simulink model "svpwm_matlab"  (Simulink 7.4)
settings: Solver=ode45  StartTime=0.0  StopTime=0.4  RelTol=1e-3
InitFcn:
  | fc_bus=50;
  | car_freq=4500;
  | TsMLIV=20e-6;
  | Ts=2e-6;
undefined symbols (not defined in the file): DiscIntNeverNeededParam
libraries: powerlib x15, powerlib_extras x3, AC2DriveInternalModels x2
settings Model: Creator=Kashif  LastModifiedBy=Kashif

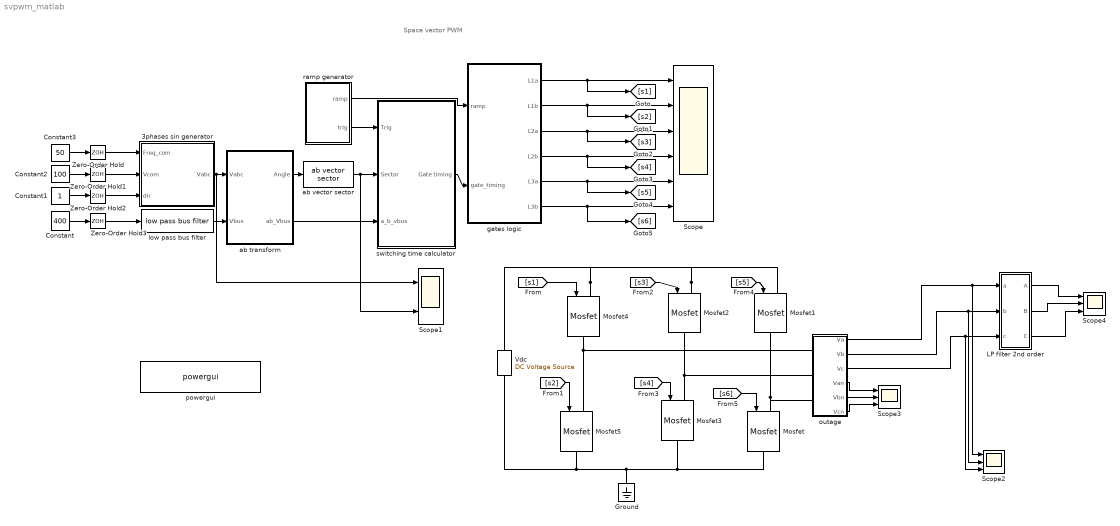
== system svpwm_matlab ==
  note: Space vector PWM
  3phases sin generator : Subsystem  AncestorBlock=AC2DriveInternalModels/SVM generator/3phases sin generator
  Constant : Constant  Value=400  OutDataType=fixdt(1, 16)  OutScaling=2^0
  Constant1 : Constant  OutDataType=fixdt(1, 16)  OutScaling=2^0
  Constant2 : Constant  Value=100  OutDataType=fixdt(1, 16)  OutScaling=2^0
  Constant3 : Constant  Value=50  OutDataType=fixdt(1, 16)  OutScaling=2^0
  Ground : powerlib/Elements/Ground  DialogController=POWERSYS.PowerSysDialog  PhysicalDomain=powersysdomain  SubClassName=unknown  LeftPortType=p1  RightPortType=p1  LConnTagsString=a
  LP filter 2nd order : Subsystem  mask{cutoff_frequency=200, damping_factor=0.707}
      mask prompts: cutoff_frequency "Cut off frequency"; damping_factor "Damping Factor"
  Mosfet{,1..5} (6 alike) : powerlib/Power Electronics/Mosfet  DialogController=POWERSYS.PowerSysDialog  SystemSampleTime=-1  Ron=0.1  Lon=0  Rd=0.01  Vfd=0  IC=0  Rs=1e5  Cs=inf  Measurements=off
  Scope : Scope  NumInputPorts=6
      settings: YMin=-5~-5~-5~-5~-5~-5  YMax=5~5~5~5~5~5  MaxDataPoints=5000000  SampleInput=on  SampleTime=2e-6
  Scope1 : Scope  NumInputPorts=2
      settings: YMin=-5~-5  YMax=5~5  MaxDataPoints=5000000  SampleInput=on  SampleTime=2e-6
  Scope2 : Scope  NumInputPorts=3
      settings: YMin=-450~-5~-5  YMax=450~5~5  SaveName=Line_voltages  MaxDataPoints=5000000  SampleInput=on  SampleTime=2e-6
  Scope3 : Scope  NumInputPorts=3
      settings: YMin=-5~-5~-5  YMax=5~5~5  SaveName=Neutral_voltages  MaxDataPoints=5000000  SampleInput=on  SampleTime=2e-6
  Scope4 : Scope  NumInputPorts=3
      settings: YMin=-450~-450~-450  YMax=450~450~450  SaveName=Filtered_voltages  MaxDataPoints=5000000  SampleInput=on  SampleTime=2e-6
  Vdc : powerlib/Electrical Sources/DC Voltage Source  DialogController=POWERSYS.PowerSysDialog  SystemSampleTime=-1  Amplitude=400  Measurements=None
  Zero-Order Hold{,1..3} (4 alike) : ZeroOrderHold  SampleTime=TsMLIV
  ab transform : Subsystem  AncestorBlock=AC2DriveInternalModels/SVM generator/ab transform
  ab vector sector : AC2DriveInternalModels/SVM generator/ab vector sector  SystemSampleTime=-1
  gates logic : Subsystem  AncestorBlock=AC2DriveInternalModels/SVM generator/gates logic
  low pass bus filter : AC2DriveInternalModels/SVM generator/low pass bus filter  SystemSampleTime=-1
  outage : Subsystem
  powergui : powerlib/powergui  Priority=1  SystemSampleTime=-1  SimulationMode=Discrete  SampleTime=2e-6  frequency=60  SPID=off  DisableSnubberDevices=off  DisableRonSwitches=off  DisableVfSwitches=off  SwTol=0  Interpol=off  frequencyindice=0  echomessages=off  HookPort=off  DisplayEquations=off  FunctionMessages=off  EnableUseOfTLC=off  x0status=blocks  RestoreLinks=warning  Frange=[0:2:500]  Ylog=off  Xlog=on  ShowGrid=off  save=off  variable=ZData  structure=Line_voltages  ZoomFFT=off  StartTime=0.04  cycles=1  DisplayStyle=2  fundamental=50  FreqAxis=off  MaxFrequency=10000  frequencyindicesteady=1  RmsSteady=1  display=off  Ts=0  methode=off
  ramp generator : Subsystem  AncestorBlock=AC2DriveInternalModels/SVM generator/ramp generator
  switching time calculator : Subsystem  AncestorBlock=AC2DriveInternalModels/SVM generator/switching time calculator
  wires:
  Zero-Order Hold3/1 -> low pass bus filter/1
  Zero-Order Hold2/1 -> 3phases sin generator/3(dir)
  Zero-Order Hold1/1 -> 3phases sin generator/2(Vcom)
  Zero-Order Hold/1 -> 3phases sin generator/1(Freq_com)
  Constant1/1 -> Zero-Order Hold2/1
  ramp generator/2(trig) -> switching time calculator/1(Trig)
  switching time calculator/1(Gate timing) -> gates logic/2(gate_timing)
  ramp generator/1(ramp) -> gates logic/1(ramp)
  ab transform/2(ab_Vbus) -> switching time calculator/3(a_b_vbus)
  ab vector sector/1 -> switching time calculator/2(Sector), Scope1/2
  3phases sin generator/1(Vabc) -> ab transform/1(Vabc), Scope1/1
  Constant2/1 -> Zero-Order Hold1/1
  ab transform/1(Angle) -> ab vector sector/1
  low pass bus filter/1 -> ab transform/2(Vbus)
  Constant/1 -> Zero-Order Hold3/1
  Constant3/1 -> Zero-Order Hold/1
  gates logic/1(L1a) -> Scope/1, [s1]
  gates logic/2(L1b) -> Scope/2, [s2]
  gates logic/3(L2a) -> Scope/3, [s3]
  gates logic/4(L2b) -> Scope/4, [s4]
  gates logic/5(L3a) -> Scope/5, [s5]
  gates logic/6(L3b) -> Scope/6, [s6]
  [s1] -> Mosfet4/1
  [s2] -> Mosfet5/1
  [s3] -> Mosfet2/1
  [s4] -> Mosfet3/1
  [s5] -> Mosfet1/1
  [s6] -> Mosfet/1
  outage/1(Va) -> Scope2/1, LP filter 2nd order/1(a)
  outage/2(Vb) -> Scope2/2, LP filter 2nd order/2(b)
  outage/3(Vc) -> Scope2/3, LP filter 2nd order/3(c)
  outage/4(Van) -> Scope3/1
  outage/5(Vbn) -> Scope3/2
  outage/6(Vcn) -> Scope3/3
  LP filter 2nd order/1(A) -> Scope4/1
  LP filter 2nd order/2(B) -> Scope4/2
  LP filter 2nd order/3(C) -> Scope4/3
  connections:
  Vdc/RConn1 -- Mosfet4/LConn1 -- Mosfet2/LConn1 -- Mosfet1/LConn1
  outage/LConn1 -- Mosfet4/RConn1 -- Mosfet5/LConn1
  outage/LConn3 -- Mosfet/LConn1 -- Mosfet1/RConn1
  Ground/LConn1 -- Mosfet/RConn1 -- Mosfet3/RConn1 -- Vdc/LConn1 -- Mosfet5/RConn1
  Mosfet3/LConn1 -- outage/LConn2 -- Mosfet2/RConn1

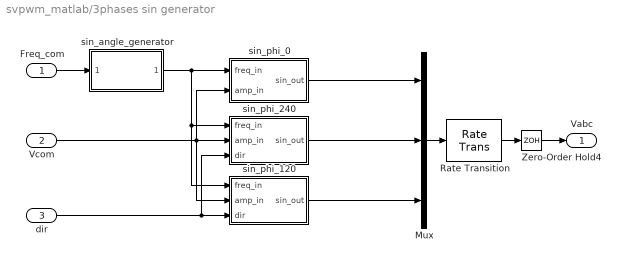
== system svpwm_matlab/3phases sin generator ==
  Freq_com : Inport  OutDataType=sfix(16)  OutScaling=2^0
  Vcom : Inport  Port=2  OutDataType=sfix(16)  OutScaling=2^0
  dir : Inport  Port=3  OutDataType=sfix(16)  OutScaling=2^0
  Mux : Mux  Inputs=3
  Rate Transition : RateTransition
  Zero-Order Hold4 : ZeroOrderHold  SampleTime=Ts
  sin_angle_generator : Subsystem
  sin_phi_0 : Subsystem
  sin_phi_120 : Subsystem
  sin_phi_240 : Subsystem
  Vabc : Outport  OutDataType=sfix(16)  OutScaling=2^0
  wires:
  Zero-Order Hold4/1 -> Vabc/1
  Mux/1 -> Rate Transition/1
  Rate Transition/1 -> Zero-Order Hold4/1
  dir/1 -> sin_phi_240/3(dir), sin_phi_120/3(dir)
  Vcom/1 -> sin_phi_120/2(amp_in), sin_phi_240/2(amp_in), sin_phi_0/2(amp_in)
  Freq_com/1 -> sin_angle_generator/1(freq_in)
  sin_angle_generator/1(sin_out) -> sin_phi_120/1(freq_in), sin_phi_240/1(freq_in), sin_phi_0/1(freq_in)
  sin_phi_120/1(sin_out) -> Mux/3
  sin_phi_240/1(sin_out) -> Mux/2
  sin_phi_0/1(sin_out) -> Mux/1

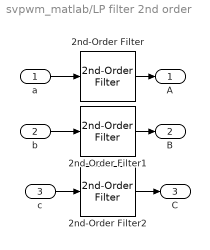
== system svpwm_matlab/LP filter 2nd order ==
  a : Inport  OutDataType=sfix(16)  OutScaling=2^0
  b : Inport  Port=2  OutDataType=sfix(16)  OutScaling=2^0
  c : Inport  Port=3  OutDataType=sfix(16)  OutScaling=2^0
  2nd-Order Filter : powerlib_extras/Control  Blocks/2nd-Order Filter  DialogController=POWERSYS.PowerSysDialog  SystemSampleTime=-1  FilterType=Lowpass  Fo=cutoff_frequency  Zeta=damping_factor  Initialize=off  Vac_Init=[1 45 60]  Vdc_Init=-0.5  PlotResponse=off  param1=[1 500 1]
  2nd-Order Filter1 : powerlib_extras/Control  Blocks/2nd-Order Filter  DialogController=POWERSYS.PowerSysDialog  SystemSampleTime=-1  FilterType=Lowpass  Fo=cutoff_frequency  Zeta=damping_factor  Initialize=off  Vac_Init=[1 45 60]  Vdc_Init=-0.5  PlotResponse=off  param1=[1 500 1]
  2nd-Order Filter2 : powerlib_extras/Control  Blocks/2nd-Order Filter  DialogController=POWERSYS.PowerSysDialog  SystemSampleTime=-1  FilterType=Lowpass  Fo=cutoff_frequency  Zeta=damping_factor  Initialize=off  Vac_Init=[1 45 60]  Vdc_Init=-0.5  PlotResponse=off  param1=[1 500 1]
  A : Outport  OutDataType=sfix(16)  OutScaling=2^0
  B : Outport  Port=2  OutDataType=sfix(16)  OutScaling=2^0
  C : Outport  Port=3  OutDataType=sfix(16)  OutScaling=2^0
  wires:
  a/1 -> 2nd-Order Filter/1
  2nd-Order Filter/1 -> A/1
  b/1 -> 2nd-Order Filter1/1
  2nd-Order Filter1/1 -> B/1
  c/1 -> 2nd-Order Filter2/1
  2nd-Order Filter2/1 -> C/1

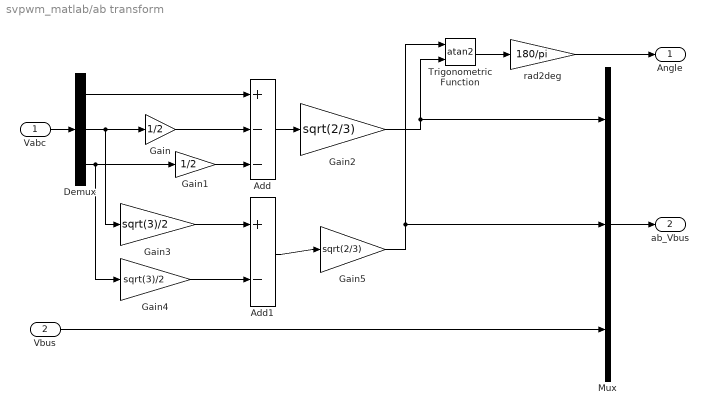
== system svpwm_matlab/ab transform ==
  Vabc : Inport  OutDataType=sfix(16)  OutScaling=2^0
  Vbus : Inport  Port=2  OutDataType=sfix(16)  OutScaling=2^0
  Add : Sum  Inputs=+--  OutDataType=fixdt(1, 16)  OutScaling=2^-10
  Add1 : Sum  Inputs=+-  OutDataType=fixdt(1, 16)  OutScaling=2^-10
  Demux : Demux  Outputs=3
  Gain : Gain  Gain=1/2  ParameterDataType=sfix(16)  ParameterScaling=2^0  OutDataType=sfix(16)  OutScaling=2^0  SaturateOnIntegerOverflow=on  OutDataTypeStr=Inherit: Same as input  ParamDataTypeStr=Inherit: Same as input
  Gain1 : Gain  Gain=1/2  ParameterDataType=sfix(16)  ParameterScaling=2^0  OutDataType=sfix(16)  OutScaling=2^0  SaturateOnIntegerOverflow=on  OutDataTypeStr=Inherit: Same as input  ParamDataTypeStr=Inherit: Same as input
  Gain2 : Gain  Gain=sqrt(2/3)  ParameterDataType=sfix(16)  ParameterScaling=2^0  OutDataType=sfix(16)  OutScaling=2^0  SaturateOnIntegerOverflow=on  OutDataTypeStr=Inherit: Same as input  ParamDataTypeStr=Inherit: Same as input
  Gain3 : Gain  Gain=sqrt(3)/2  ParameterDataType=sfix(16)  ParameterScaling=2^0  OutDataType=sfix(16)  OutScaling=2^0  SaturateOnIntegerOverflow=on  OutDataTypeStr=Inherit: Same as input  ParamDataTypeStr=Inherit: Same as input
  Gain4 : Gain  Gain=sqrt(3)/2  ParameterDataType=sfix(16)  ParameterScaling=2^0  OutDataType=sfix(16)  OutScaling=2^0  SaturateOnIntegerOverflow=on  OutDataTypeStr=Inherit: Same as input  ParamDataTypeStr=Inherit: Same as input
  Gain5 : Gain  Gain=sqrt(2/3)  ParameterDataType=sfix(16)  ParameterScaling=2^0  OutDataType=sfix(16)  OutScaling=2^0  SaturateOnIntegerOverflow=on  OutDataTypeStr=Inherit: Same as input  ParamDataTypeStr=Inherit: Same as input
  Mux : Mux  Inputs=3
  Trigonometric Function : Trigonometry  Operator=atan2
  rad2deg : Gain  Gain=180/pi  ParameterDataType=sfix(16)  ParameterScaling=2^0  OutDataType=sfix(16)  OutScaling=2^0  SaturateOnIntegerOverflow=on  OutDataTypeStr=Inherit: Same as input  ParamDataTypeStr=Inherit: Same as input
  Angle : Outport  OutDataType=sfix(16)  OutScaling=2^0
  ab_Vbus : Outport  Port=2  OutDataType=sfix(16)  OutScaling=2^0
  wires:
  Gain2/1 -> Mux/1, Trigonometric Function/2
  Trigonometric Function/1 -> rad2deg/1
  Mux/1 -> ab_Vbus/1
  Gain5/1 -> Mux/2, Trigonometric Function/1
  Vbus/1 -> Mux/3
  rad2deg/1 -> Angle/1
  Vabc/1 -> Demux/1
  Demux/2 -> Gain/1, Gain3/1
  Demux/3 -> Gain1/1, Gain4/1
  Add/1 -> Gain2/1
  Demux/1 -> Add/1
  Gain/1 -> Add/2
  Gain1/1 -> Add/3
  Gain3/1 -> Add1/1
  Gain4/1 -> Add1/2
  Add1/1 -> Gain5/1

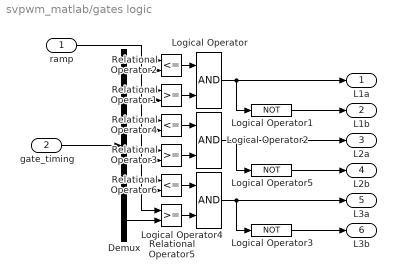
== system svpwm_matlab/gates logic ==
  ramp : Inport  OutDataType=sfix(16)  OutScaling=2^0
  gate_timing : Inport  Port=2  OutDataType=sfix(16)  OutScaling=2^0
  Demux : Demux  Outputs=6
  Logical Operator : Logic
  Logical Operator1 : Logic  Operator=NOT
  Logical Operator2 : Logic
  Logical Operator3 : Logic  Operator=NOT
  Logical Operator4 : Logic
  Logical Operator5 : Logic  Operator=NOT
  Relational Operator1 : RelationalOperator  InputSameDT=on
  Relational Operator2 : RelationalOperator  Operator=<=  InputSameDT=on
  Relational Operator3 : RelationalOperator  InputSameDT=on
  Relational Operator4 : RelationalOperator  Operator=<=  InputSameDT=on
  Relational Operator5 : RelationalOperator  InputSameDT=on
  Relational Operator6 : RelationalOperator  Operator=<=  InputSameDT=on
  L1a : Outport  OutDataType=fixdt(1, 16)  OutScaling=2^0
  L1b : Outport  Port=2  OutDataType=fixdt(1, 16)  OutScaling=2^0
  L2a : Outport  Port=3  OutDataType=fixdt(1, 16)  OutScaling=2^0
  L2b : Outport  Port=4  OutDataType=fixdt(1, 16)  OutScaling=2^0
  L3a : Outport  Port=5  OutDataType=fixdt(1, 16)  OutScaling=2^0
  L3b : Outport  Port=6  OutDataType=fixdt(1, 16)  OutScaling=2^0
  wires:
  ramp/1 -> Relational Operator2/1, Relational Operator1/1, Relational Operator4/1, Relational Operator3/1, Relational Operator6/1, Relational Operator5/1
  Relational Operator2/1 -> Logical Operator/1
  Relational Operator1/1 -> Logical Operator/2
  Relational Operator4/1 -> Logical Operator2/1
  Relational Operator3/1 -> Logical Operator2/2
  Relational Operator6/1 -> Logical Operator4/1
  Relational Operator5/1 -> Logical Operator4/2
  Logical Operator/1 -> Logical Operator1/1, L1a/1
  Logical Operator1/1 -> L1b/1
  Logical Operator2/1 -> Logical Operator5/1, L2a/1
  Logical Operator5/1 -> L2b/1
  Logical Operator4/1 -> Logical Operator3/1, L3a/1
  Logical Operator3/1 -> L3b/1
  Demux/1 -> Relational Operator2/2
  Demux/6 -> Relational Operator5/2
  Demux/5 -> Relational Operator6/2
  Demux/4 -> Relational Operator3/2
  Demux/3 -> Relational Operator4/2
  Demux/2 -> Relational Operator1/2
  gate_timing/1 -> Demux/1

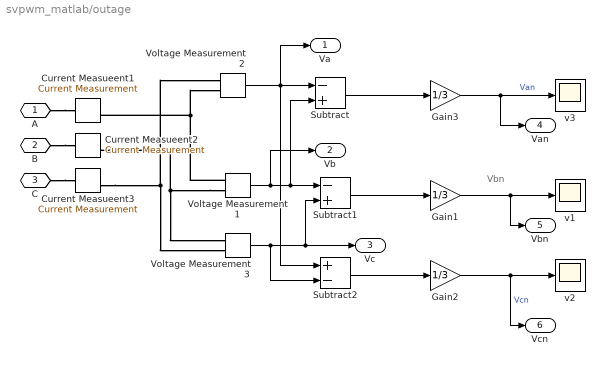
== system svpwm_matlab/outage ==
  note: Vbn
  Current Measueent1 : powerlib/Measurements/Current Measurement  DialogController=POWERSYS.PowerSysDialog  SystemSampleTime=-1  PhasorSimulation=off  OutputType=Complex  PSBequivalent=0
  Current Measueent2 : powerlib/Measurements/Current Measurement  DialogController=POWERSYS.PowerSysDialog  SystemSampleTime=-1  PhasorSimulation=off  OutputType=Complex  PSBequivalent=0
  Current Measueent3 : powerlib/Measurements/Current Measurement  DialogController=POWERSYS.PowerSysDialog  SystemSampleTime=-1  PhasorSimulation=off  OutputType=Complex  PSBequivalent=0
  Gain1 : Gain  Gain=1/3  ParameterDataType=sfix(16)  ParameterScaling=2^0  OutDataType=sfix(16)  OutScaling=2^0
  Gain2 : Gain  Gain=1/3  ParameterDataType=sfix(16)  ParameterScaling=2^0  OutDataType=sfix(16)  OutScaling=2^0
  Gain3 : Gain  Gain=1/3  ParameterDataType=sfix(16)  ParameterScaling=2^0  OutDataType=sfix(16)  OutScaling=2^0
  Subtract : Sum  Inputs=-+  OutDataType=sfix(16)  OutScaling=2^-10
  Subtract1 : Sum  Inputs=-+  OutDataType=sfix(16)  OutScaling=2^-10
  Subtract2 : Sum  Inputs=+-  OutDataType=sfix(16)  OutScaling=2^-10
  Voltage Measurement1 : powerlib/Measurements/Voltage Measurement  DialogController=POWERSYS.PowerSysDialog  SystemSampleTime=-1  PhasorSimulation=off  OutputType=Complex  PSBequivalent=0
  Voltage Measurement2 : powerlib/Measurements/Voltage Measurement  DialogController=POWERSYS.PowerSysDialog  SystemSampleTime=-1  PhasorSimulation=off  OutputType=Complex  PSBequivalent=0
  Voltage Measurement3 : powerlib/Measurements/Voltage Measurement  DialogController=POWERSYS.PowerSysDialog  SystemSampleTime=-1  PhasorSimulation=off  OutputType=Complex  PSBequivalent=0
  v1 : Scope
      settings: SaveName=ScopeData25  MaxDataPoints=5000000
  v2 : Scope
      settings: SaveName=ScopeData26  MaxDataPoints=5000000
  v3 : Scope
      settings: YMin=-300  YMax=300  SaveName=ScopeData27  MaxDataPoints=5000000
  A : PMIOPort  Port=1  Side=Left
  B : PMIOPort  Port=2  Side=Left
  C : PMIOPort  Port=3  Side=Left
  Va : Outport  OutDataType=sfix(16)  OutScaling=2^0
  Vb : Outport  Port=2  OutDataType=sfix(16)  OutScaling=2^0
  Vc : Outport  Port=3  OutDataType=sfix(16)  OutScaling=2^0
  Van : Outport  Port=4  OutDataType=sfix(16)  OutScaling=2^0
  Vbn : Outport  Port=5  OutDataType=sfix(16)  OutScaling=2^0
  Vcn : Outport  Port=6  OutDataType=sfix(16)  OutScaling=2^0
  wires:
  Gain2/1 -> v2/1, Vcn/1  "Vcn"
  Subtract2/1 -> Gain2/1
  Gain1/1 -> v1/1, Vbn/1
  Subtract1/1 -> Gain1/1
  Voltage Measurement3/1 -> Subtract2/2, Subtract1/2, Vc/1
  Gain3/1 -> v3/1, Van/1  "Van"
  Subtract/1 -> Gain3/1
  Voltage Measurement1/1 -> Subtract/2, Subtract1/1, Vb/1
  Voltage Measurement2/1 -> Subtract/1, Subtract2/1, Va/1
  connections:
  Voltage Measurement1/LConn1 -- Current Measueent1/RConn1 -- Voltage Measurement2/LConn2
  Voltage Measurement1/LConn2 -- Current Measueent2/RConn1 -- Voltage Measurement3/LConn1
  Current Measueent3/RConn1 -- Voltage Measurement2/LConn1 -- Voltage Measurement3/LConn2
  A/RConn1 -- Current Measueent1/LConn1
  B/RConn1 -- Current Measueent2/LConn1
  C/RConn1 -- Current Measueent3/LConn1

== system svpwm_matlab/ramp generator ==
  Constant3 : Constant  OutDataType=sfix(16)  OutScaling=2^0
  Discrete-Time Integrator1 : DiscreteIntegrator  ExternalReset=rising  SampleTime=Ts  OutDataType=sfix(16)  OutScaling=2^0  ICPrevOutput=DiscIntNeverNeededParam  ICPrevScaledInput=DiscIntNeverNeededParam
  Relational Operator1 : RelationalOperator  InputSameDT=on
  Scope : Scope
      settings: SaveName=ScopeData2  MaxDataPoints=5000000  SampleInput=on  SampleTime=2e-6
  Unit Delay1 : UnitDelay  SampleTime=Ts
  fc : Constant  Value=car_freq  OutDataType=sfix(16)  OutScaling=2^0
  ramp : Outport  OutDataType=sfix(16)  OutScaling=2^0
  trig : Outport  Port=2  OutDataType=sfix(16)  OutScaling=2^0
  wires:
  fc/1 -> Discrete-Time Integrator1/1
  Discrete-Time Integrator1/1 -> Relational Operator1/1, ramp/1, Scope/1
  Constant3/1 -> Relational Operator1/2
  Relational Operator1/1 -> Unit Delay1/1
  Unit Delay1/1 -> Discrete-Time Integrator1/2, trig/1

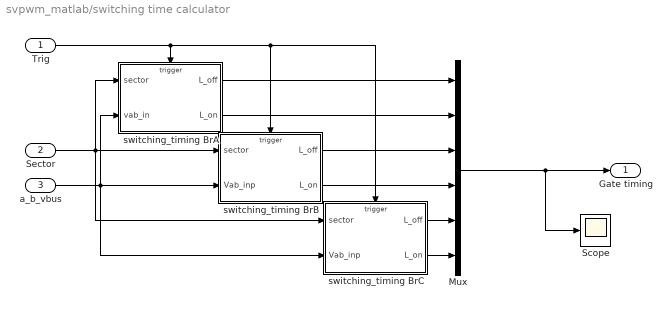
== system svpwm_matlab/switching time calculator ==
  Trig : Inport  OutDataType=sfix(16)  OutScaling=2^0
  Sector : Inport  Port=2  OutDataType=sfix(16)  OutScaling=2^0
  a_b_vbus : Inport  Port=3  OutDataType=sfix(16)  OutScaling=2^0
  Mux : Mux  Inputs=6
  Scope : Scope
      settings: YMax=6  SaveName=ScopeData3  MaxDataPoints=5000000  SampleInput=on  SampleTime=2e-6
  switching_timing BrA : Subsystem  TreatAsAtomicUnit=on
  switching_timing BrB : Subsystem  TreatAsAtomicUnit=on
  switching_timing BrC : Subsystem  TreatAsAtomicUnit=on
  Gate timing : Outport  OutDataType=sfix(16)  OutScaling=2^0
  wires:
  switching_timing BrA/1(L_off) -> Mux/1
  switching_timing BrA/2(L_on) -> Mux/2
  switching_timing BrB/1(L_off) -> Mux/3
  switching_timing BrB/2(L_on) -> Mux/4
  switching_timing BrC/1(L_off) -> Mux/5
  switching_timing BrC/2(L_on) -> Mux/6
  Sector/1 -> switching_timing BrB/1(sector), switching_timing BrC/1(sector), switching_timing BrA/1(sector)
  a_b_vbus/1 -> switching_timing BrB/2(Vab_inp), switching_timing BrA/2(vab_in), switching_timing BrC/2(Vab_inp)
  Trig/1 -> switching_timing BrA/Trigger, switching_timing BrB/Trigger, switching_timing BrC/Trigger
  Mux/1 -> Gate timing/1, Scope/1

== system svpwm_matlab/3phases sin generator/sin_angle_generator ==
  freq_in : Inport  OutDataType=sfix(16)  OutScaling=2^0
  Constant : Constant  Value=360  OutDataType=sfix(16)  OutScaling=2^0
  Constant1 : Constant  Value=360  OutDataType=sfix(16)  OutScaling=2^0
  Discrete-Time Integrator : DiscreteIntegrator  IntegratorMethod=Integration: Trapezoidal  ExternalReset=rising  SampleTime=TsMLIV  OutDataType=sfix(16)  OutScaling=2^0  ICPrevOutput=DiscIntNeverNeededParam  ICPrevScaledInput=DiscIntNeverNeededParam
  Product : Product  OutDataType=sfix(16)  OutScaling=2^0  SaturateOnIntegerOverflow=on  InputSameDT=on  OutDataTypeStr=Inherit: Same as first input
  Relational Operator : RelationalOperator  InputSameDT=on
  Unit Delay : UnitDelay  SampleTime=TsMLIV
  sin_out : Outport  OutDataType=sfix(16)  OutScaling=2^0
  wires:
  Unit Delay/1 -> Discrete-Time Integrator/2
  Relational Operator/1 -> Unit Delay/1
  Constant1/1 -> Relational Operator/2
  Discrete-Time Integrator/1 -> Relational Operator/1, sin_out/1
  freq_in/1 -> Product/2
  Constant/1 -> Product/1
  Product/1 -> Discrete-Time Integrator/1

== system svpwm_matlab/3phases sin generator/sin_phi_0 ==
  freq_in : Inport  OutDataType=sfix(16)  OutScaling=2^0
  amp_in : Inport  Port=2  OutDataType=sfix(16)  OutScaling=2^0
  Product : Product  OutDataType=sfix(16)  OutScaling=2^0  SaturateOnIntegerOverflow=on  InputSameDT=on  OutDataTypeStr=Inherit: Same as first input
  Trigonometric Function : Trigonometry
  d2r : Gain  Gain=pi/180  ParameterDataType=sfix(16)  ParameterScaling=2^0  OutDataType=sfix(16)  OutScaling=2^0  SaturateOnIntegerOverflow=on  OutDataTypeStr=Inherit: Same as input  ParamDataTypeStr=Inherit: Same as input
  sin_out : Outport  OutDataType=sfix(16)  OutScaling=2^0
  wires:
  Product/1 -> sin_out/1
  amp_in/1 -> Product/2
  Trigonometric Function/1 -> Product/1
  d2r/1 -> Trigonometric Function/1
  freq_in/1 -> d2r/1

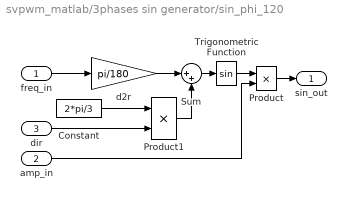
== system svpwm_matlab/3phases sin generator/sin_phi_120 ==
  freq_in : Inport  OutDataType=sfix(16)  OutScaling=2^0
  amp_in : Inport  Port=2  OutDataType=sfix(16)  OutScaling=2^0
  dir : Inport  Port=3  OutDataType=sfix(16)  OutScaling=2^0
  Constant : Constant  Value=2*pi/3  OutDataType=sfix(16)  OutScaling=2^0
  Product : Product  OutDataType=sfix(16)  OutScaling=2^0  SaturateOnIntegerOverflow=on  InputSameDT=on  OutDataTypeStr=Inherit: Same as first input
  Product1 : Product  OutDataType=sfix(16)  OutScaling=2^0  SaturateOnIntegerOverflow=on  InputSameDT=on  OutDataTypeStr=Inherit: Same as first input
  Sum : Sum  Inputs=|++  OutDataType=sfix(16)  OutScaling=2^0  SaturateOnIntegerOverflow=on  InputSameDT=on  OutDataTypeStr=Inherit: Same as first input
  Trigonometric Function : Trigonometry
  d2r : Gain  Gain=pi/180  ParameterDataType=sfix(16)  ParameterScaling=2^0  OutDataType=sfix(16)  OutScaling=2^0  SaturateOnIntegerOverflow=on  OutDataTypeStr=Inherit: Same as input  ParamDataTypeStr=Inherit: Same as input
  sin_out : Outport  OutDataType=sfix(16)  OutScaling=2^0
  wires:
  freq_in/1 -> d2r/1
  Trigonometric Function/1 -> Product/1
  amp_in/1 -> Product/2
  Product/1 -> sin_out/1
  Sum/1 -> Trigonometric Function/1
  d2r/1 -> Sum/1
  dir/1 -> Product1/2
  Constant/1 -> Product1/1
  Product1/1 -> Sum/2

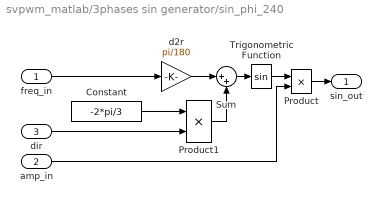
== system svpwm_matlab/3phases sin generator/sin_phi_240 ==
  freq_in : Inport  OutDataType=sfix(16)  OutScaling=2^0
  amp_in : Inport  Port=2  OutDataType=sfix(16)  OutScaling=2^0
  dir : Inport  Port=3  OutDataType=sfix(16)  OutScaling=2^0
  Constant : Constant  Value=-2*pi/3  OutDataType=sfix(16)  OutScaling=2^0
  Product : Product  OutDataType=sfix(16)  OutScaling=2^0  SaturateOnIntegerOverflow=on  InputSameDT=on  OutDataTypeStr=Inherit: Same as first input
  Product1 : Product  OutDataType=sfix(16)  OutScaling=2^0  SaturateOnIntegerOverflow=on  InputSameDT=on  OutDataTypeStr=Inherit: Same as first input
  Sum : Sum  Inputs=|++  OutDataType=sfix(16)  OutScaling=2^0  SaturateOnIntegerOverflow=on  InputSameDT=on  OutDataTypeStr=Inherit: Same as first input
  Trigonometric Function : Trigonometry
  d2r : Gain  Gain=pi/180  ParameterDataType=sfix(16)  ParameterScaling=2^0  OutDataType=sfix(16)  OutScaling=2^0  SaturateOnIntegerOverflow=on  OutDataTypeStr=Inherit: Same as input  ParamDataTypeStr=Inherit: Same as input
  sin_out : Outport  OutDataType=sfix(16)  OutScaling=2^0
  wires:
  Product1/1 -> Sum/2
  Constant/1 -> Product1/1
  dir/1 -> Product1/2
  d2r/1 -> Sum/1
  Sum/1 -> Trigonometric Function/1
  Product/1 -> sin_out/1
  amp_in/1 -> Product/2
  Trigonometric Function/1 -> Product/1
  freq_in/1 -> d2r/1

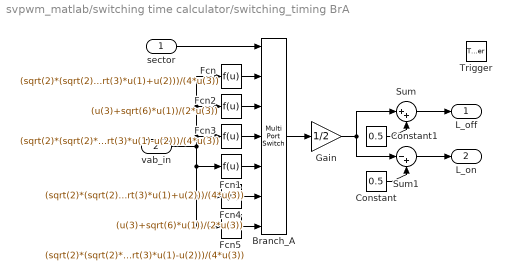
== system svpwm_matlab/switching time calculator/switching_timing BrA ==
  sector : Inport  OutDataType=sfix(16)  OutScaling=2^0
  vab_in : Inport  Port=2  OutDataType=sfix(16)  OutScaling=2^0
  Trigger : TriggerPort
  Branch_A : MultiPortSwitch  Inputs=6  SaturateOnIntegerOverflow=on  InputSameDT=on
  Constant : Constant  Value=0.5  OutDataType=sfix(16)  OutScaling=2^0
  Constant1 : Constant  Value=0.5  OutDataType=sfix(16)  OutScaling=2^0
  Fcn : Fcn  Expr=(sqrt(2)*(sqrt(2)*u(3)+sqrt(3)*u(1)+u(2)))/(4*u(3))
  Fcn1 : Fcn  Expr=(sqrt(2)*(sqrt(2)*u(3)+sqrt(3)*u(1)+u(2)))/(4*u(3))
  Fcn2 : Fcn  Expr=(u(3)+sqrt(6)*u(1))/(2*u(3))
  Fcn3 : Fcn  Expr=(sqrt(2)*(sqrt(2)*u(3)+sqrt(3)*u(1)-u(2)))/(4*u(3))
  Fcn4 : Fcn  Expr=(u(3)+sqrt(6)*u(1))/(2*u(3))
  Fcn5 : Fcn  Expr=(sqrt(2)*(sqrt(2)*u(3)+sqrt(3)*u(1)-u(2)))/(4*u(3))
  Gain : Gain  Gain=1/2  ParameterDataType=sfix(16)  ParameterScaling=2^0  OutDataType=sfix(16)  OutScaling=2^0  SaturateOnIntegerOverflow=on  OutDataTypeStr=Inherit: Same as input  ParamDataTypeStr=Inherit: Same as input
  Sum : Sum  Inputs=|++  OutDataType=sfix(16)  OutScaling=2^0  SaturateOnIntegerOverflow=on  InputSameDT=on  OutDataTypeStr=Inherit: Same as first input
  Sum1 : Sum  Inputs=|-+  OutDataType=sfix(16)  OutScaling=2^0  SaturateOnIntegerOverflow=on  InputSameDT=on  OutDataTypeStr=Inherit: Same as first input
  L_off : Outport  OutDataType=sfix(16)  OutScaling=2^0
  L_on : Outport  Port=2  OutDataType=sfix(16)  OutScaling=2^0
  wires:
  Fcn/1 -> Branch_A/2
  Fcn2/1 -> Branch_A/3
  Fcn3/1 -> Branch_A/4
  Fcn1/1 -> Branch_A/5
  Fcn4/1 -> Branch_A/6
  Fcn5/1 -> Branch_A/7
  Branch_A/1 -> Gain/1
  Gain/1 -> Sum/1, Sum1/1
  Constant/1 -> Sum1/2
  Constant1/1 -> Sum/2
  Sum/1 -> L_off/1
  Sum1/1 -> L_on/1
  sector/1 -> Branch_A/1
  vab_in/1 -> Fcn3/1, Fcn2/1, Fcn/1, Fcn1/1, Fcn4/1, Fcn5/1

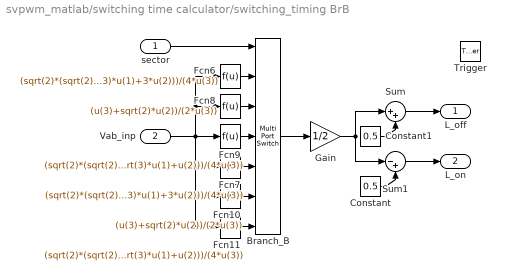
== system svpwm_matlab/switching time calculator/switching_timing BrB ==
  sector : Inport  OutDataType=sfix(16)  OutScaling=2^0
  Vab_inp : Inport  Port=2  OutDataType=sfix(16)  OutScaling=2^0
  Trigger : TriggerPort
  Branch_B : MultiPortSwitch  Inputs=6  SaturateOnIntegerOverflow=on  InputSameDT=on
  Constant : Constant  Value=0.5  OutDataType=sfix(16)  OutScaling=2^0
  Constant1 : Constant  Value=0.5  OutDataType=sfix(16)  OutScaling=2^0
  Fcn10 : Fcn  Expr=(u(3)+sqrt(2)*u(2))/(2*u(3))
  Fcn11 : Fcn  Expr=(sqrt(2)*(sqrt(2)*u(3)-sqrt(3)*u(1)+u(2)))/(4*u(3))
  Fcn6 : Fcn  Expr=(sqrt(2)*(sqrt(2)*u(3)-sqrt(3)*u(1)+3*u(2)))/(4*u(3))
  Fcn7 : Fcn  Expr=(sqrt(2)*(sqrt(2)*u(3)-sqrt(3)*u(1)+3*u(2)))/(4*u(3))
  Fcn8 : Fcn  Expr=(u(3)+sqrt(2)*u(2))/(2*u(3))
  Fcn9 : Fcn  Expr=(sqrt(2)*(sqrt(2)*u(3)-sqrt(3)*u(1)+u(2)))/(4*u(3))
  Gain : Gain  Gain=1/2  ParameterDataType=sfix(16)  ParameterScaling=2^0  OutDataType=sfix(16)  OutScaling=2^0  SaturateOnIntegerOverflow=on  OutDataTypeStr=Inherit: Same as input  ParamDataTypeStr=Inherit: Same as input
  Sum : Sum  Inputs=|++  OutDataType=sfix(16)  OutScaling=2^0  SaturateOnIntegerOverflow=on  InputSameDT=on  OutDataTypeStr=Inherit: Same as first input
  Sum1 : Sum  Inputs=|-+  OutDataType=sfix(16)  OutScaling=2^0  SaturateOnIntegerOverflow=on  InputSameDT=on  OutDataTypeStr=Inherit: Same as first input
  L_off : Outport  OutDataType=sfix(16)  OutScaling=2^0
  L_on : Outport  Port=2  OutDataType=sfix(16)  OutScaling=2^0
  wires:
  sector/1 -> Branch_B/1
  Sum1/1 -> L_on/1
  Sum/1 -> L_off/1
  Constant1/1 -> Sum/2
  Constant/1 -> Sum1/2
  Gain/1 -> Sum1/1, Sum/1
  Branch_B/1 -> Gain/1
  Vab_inp/1 -> Fcn10/1, Fcn11/1, Fcn7/1, Fcn8/1, Fcn6/1, Fcn9/1
  Fcn7/1 -> Branch_B/5
  Fcn8/1 -> Branch_B/3
  Fcn6/1 -> Branch_B/2
  Fcn9/1 -> Branch_B/4
  Fcn10/1 -> Branch_B/6
  Fcn11/1 -> Branch_B/7

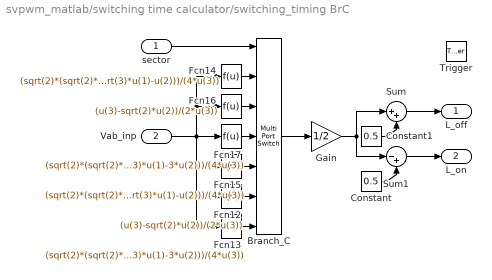
== system svpwm_matlab/switching time calculator/switching_timing BrC ==
  sector : Inport  OutDataType=sfix(16)  OutScaling=2^0
  Vab_inp : Inport  Port=2  OutDataType=sfix(16)  OutScaling=2^0
  Trigger : TriggerPort
  Branch_C : MultiPortSwitch  Inputs=6  SaturateOnIntegerOverflow=on  InputSameDT=on
  Constant : Constant  Value=0.5  OutDataType=sfix(16)  OutScaling=2^0
  Constant1 : Constant  Value=0.5  OutDataType=sfix(16)  OutScaling=2^0
  Fcn12 : Fcn  Expr=(u(3)-sqrt(2)*u(2))/(2*u(3))
  Fcn13 : Fcn  Expr=(sqrt(2)*(sqrt(2)*u(3)-sqrt(3)*u(1)-3*u(2)))/(4*u(3))
  Fcn14 : Fcn  Expr=(sqrt(2)*(sqrt(2)*u(3)-sqrt(3)*u(1)-u(2)))/(4*u(3))
  Fcn15 : Fcn  Expr=(sqrt(2)*(sqrt(2)*u(3)-sqrt(3)*u(1)-u(2)))/(4*u(3))
  Fcn16 : Fcn  Expr=(u(3)-sqrt(2)*u(2))/(2*u(3))
  Fcn17 : Fcn  Expr=(sqrt(2)*(sqrt(2)*u(3)-sqrt(3)*u(1)-3*u(2)))/(4*u(3))
  Gain : Gain  Gain=1/2  ParameterDataType=sfix(16)  ParameterScaling=2^0  OutDataType=sfix(16)  OutScaling=2^0  SaturateOnIntegerOverflow=on  OutDataTypeStr=Inherit: Same as input  ParamDataTypeStr=Inherit: Same as input
  Sum : Sum  Inputs=|++  OutDataType=sfix(16)  OutScaling=2^0  SaturateOnIntegerOverflow=on  InputSameDT=on  OutDataTypeStr=Inherit: Same as first input
  Sum1 : Sum  Inputs=|-+  OutDataType=sfix(16)  OutScaling=2^0  SaturateOnIntegerOverflow=on  InputSameDT=on  OutDataTypeStr=Inherit: Same as first input
  L_off : Outport  OutDataType=sfix(16)  OutScaling=2^0
  L_on : Outport  Port=2  OutDataType=sfix(16)  OutScaling=2^0
  wires:
  Vab_inp/1 -> Fcn16/1, Fcn14/1, Fcn12/1, Fcn13/1, Fcn15/1, Fcn17/1
  Branch_C/1 -> Gain/1
  Gain/1 -> Sum/1, Sum1/1
  Constant/1 -> Sum1/2
  Constant1/1 -> Sum/2
  Sum/1 -> L_off/1
  Sum1/1 -> L_on/1
  Fcn15/1 -> Branch_C/5
  Fcn16/1 -> Branch_C/3
  Fcn14/1 -> Branch_C/2
  Fcn17/1 -> Branch_C/4
  Fcn12/1 -> Branch_C/6
  Fcn13/1 -> Branch_C/7
  sector/1 -> Branch_C/1
